simulink model "katayamacopter_r2021b"  (R2021b)
settings: Solver=VariableStepAuto  StartTime=0.0  StopTime=50  RelTol=1e-3
values from neighbouring files (symbols this model uses):
  A_pitch = [0  1; 0  0]    [param.mat]
  A_travel = [0  1; 0  -0.0247]    [param.mat]
  B_elev = [0  0; 0.655  0]    [param.mat]
  B_pitch = [0  0; 0  0.248]    [param.mat]
  B_travel = [0  0; 0.0086  0]    [param.mat]
  C_pitch = [1  0; 0  0]    [param.mat]
  C_travel = [1  0; 0  0]    [param.mat]
  D_elev = [0  0; 0  0]    [param.mat]
  D_pitch = [0  0; 0  0]    [param.mat]
  D_travel = [0  0; 0  0]    [param.mat]
libraries: robotlib x5, mpclib x3
settings Model: VariantFading=off  Creator=marik  LastModifiedBy=marik
settings DebuggingCC: UnconnectedInputMsg=none  UnconnectedOutputMsg=none  UnconnectedLineMsg=none  UnderSpecifiedDimensionMsg=warning
settings RTWCC: DLArmComputeVersion=20.02.1

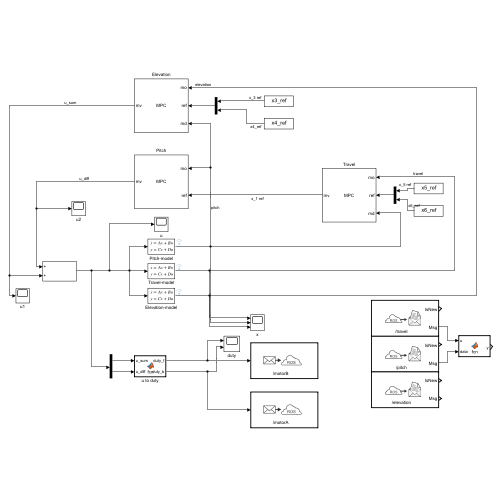
[thumbnail: Simulink's stored preview of the top-level diagram]
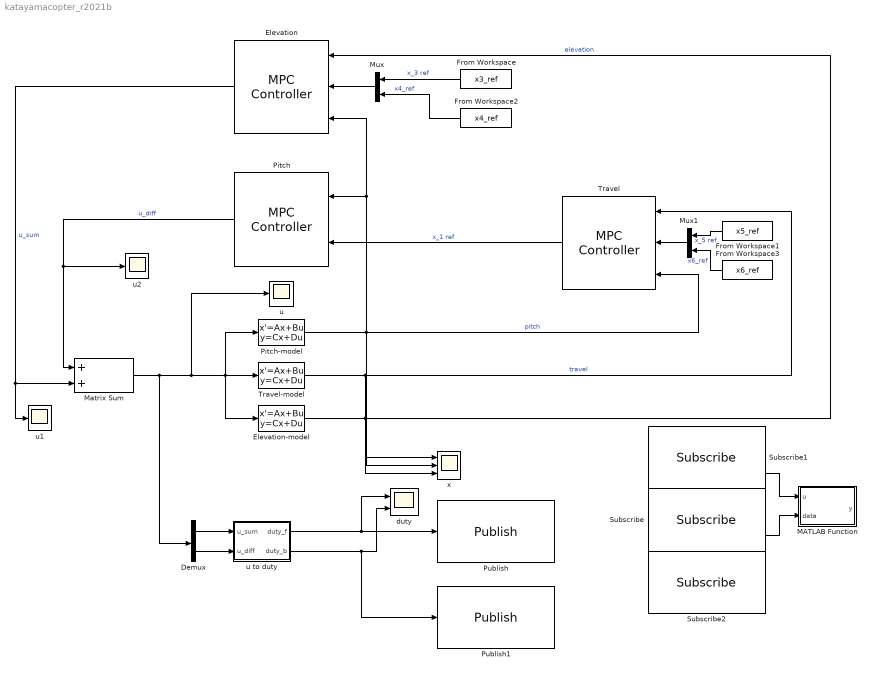
== system katayamacopter_r2021b ==
  Demux : Demux  Outputs=2
  Elevation : mpclib/MPC Controller  SCDEnableBlockLinearizationSpecification=on  mpcobj=mpcelev  is_multiple=0  enable_value=0  return_u0=off  updateMPCinCallerWorkspace=on  md_inport=on  mv_inport=off  uref_inport=off  return_cost=off  return_mvseq=off  return_qpstatus=off  return_xseq=off  return_state=off  return_ovseq=off  state_inport=off  umin_inport=off  umax_inport=off  ymin_inport=off  ymax_inport=off  cc_inport=off  ywt_inport=off  uwt_inport=off  duwt_inport=off  rhoeps_inport=off  pm_inport=off  MaximumP=10  HorizonChoice=FixedHorizon  n_ts=0.1  n_p=10  n_mv=2  n_md=1  n_ud=0  n_mo=2  n_uo=0  BlockDataType=double  SampleTimeInherited=off  switch_inport=off
  Elevation-model : StateSpace  A=[0 1;-1.283 -0.11]  B=B_elev  C=[1 0;0 1]  D=D_elev  InitialCondition=0
  From Workspace : FromWorkspace  VariableName=x3_ref  SampleTime=0.1  OutputAfterFinalValue=Holding final value
  From Workspace1 : FromWorkspace  VariableName=x5_ref  SampleTime=0.1  OutputAfterFinalValue=Holding final value
  From Workspace2 : FromWorkspace  VariableName=x4_ref
  From Workspace3 : FromWorkspace  VariableName=x6_ref
  MATLAB Function : MATLAB Function  TreatAsAtomicUnit=on
  Matrix Sum : Sum
  Mux : Mux  Inputs=2
  Mux1 : Mux  Inputs=2
  Pitch : mpclib/MPC Controller  SCDEnableBlockLinearizationSpecification=on  mpcobj=mpcpitch  is_multiple=0  enable_value=0  return_u0=off  updateMPCinCallerWorkspace=on  md_inport=off  mv_inport=off  uref_inport=off  return_cost=off  return_mvseq=off  return_qpstatus=off  return_xseq=off  return_state=off  return_ovseq=off  state_inport=off  umin_inport=off  umax_inport=off  ymin_inport=off  ymax_inport=off  cc_inport=off  ywt_inport=off  uwt_inport=off  duwt_inport=off  rhoeps_inport=off  pm_inport=off  MaximumP=10  HorizonChoice=FixedHorizon  n_ts=0.1  n_p=10  n_mv=2  n_md=0  n_ud=0  n_mo=2  n_uo=0  BlockDataType=double  SampleTimeInherited=off  switch_inport=off
  Pitch-model : StateSpace  A=A_pitch  B=B_pitch  C=C_pitch  D=D_pitch  InitialCondition=0
  Publish : robotlib/Publish  topicSource=Specify your own  topic=/motorB  messageType=std_msgs/Float32  legacyBusStruct=off  messageQueueLength=1
  Publish1 : robotlib/Publish  topicSource=Specify your own  topic=/motorA  messageType=std_msgs/Float32MultiArray  legacyBusStruct=off  messageQueueLength=1
  Subscribe : robotlib/Subscribe  topicSource=Specify your own  topic=/pitch  messageType=geometry_msgs/Point  SampleTime=-1  legacyBusStruct=off  messageQueueLength=1
  Subscribe1 : robotlib/Subscribe  topicSource=Specify your own  topic=/travel  messageType=std_msgs/Float32  SampleTime=-1  legacyBusStruct=off  messageQueueLength=1
  Subscribe2 : robotlib/Subscribe  topicSource=Specify your own  topic=/elevation  messageType=geometry_msgs/Point  SampleTime=-1  legacyBusStruct=off  messageQueueLength=1
  Travel : mpclib/MPC Controller  SCDEnableBlockLinearizationSpecification=on  mpcobj=mpctravel  is_multiple=0  enable_value=0  return_u0=off  updateMPCinCallerWorkspace=on  md_inport=on  mv_inport=off  uref_inport=off  return_cost=off  return_mvseq=off  return_qpstatus=off  return_xseq=off  return_state=off  return_ovseq=off  state_inport=off  umin_inport=off  umax_inport=off  ymin_inport=off  ymax_inport=off  cc_inport=off  ywt_inport=off  uwt_inport=off  duwt_inport=off  rhoeps_inport=off  pm_inport=off  MaximumP=10  HorizonChoice=FixedHorizon  n_ts=0.1  n_p=10  n_mv=2  n_md=1  n_ud=0  n_mo=2  n_uo=0  BlockDataType=double  SampleTimeInherited=off  switch_inport=off
  Travel-model : StateSpace  A=A_travel  B=B_travel  C=C_travel  D=D_travel  InitialCondition=0
  duty : Scope  NumInputPorts=2
  u : Scope
  u to duty : MATLAB Function  TreatAsAtomicUnit=on
  u1 : Scope
  u2 : Scope
  x : Scope  NumInputPorts=3
  wires:
  Travel/1 -> Pitch/2  "x_1 ref"
  From Workspace/1 -> Mux/1  "x_3 ref"
  Elevation-model/1 -> x/1, Elevation/1  "elevation"
  Pitch-model/1 -> x/2, Travel/3, Elevation/3, Pitch/1  "pitch"
  Travel-model/1 -> x/3, Travel/1  "travel"
  From Workspace1/1 -> Mux1/1  "x_5 ref"
  Elevation/1 -> u1/1, Matrix Sum/2  "u_sum"
  Pitch/1 -> u2/1, Matrix Sum/1  "u_diff"
  Matrix Sum/1 -> Demux/1, u/1, Pitch-model/1, Travel-model/1, Elevation-model/1
  From Workspace2/1 -> Mux/2  "x4_ref"
  Mux/1 -> Elevation/2
  Mux1/1 -> Travel/2
  From Workspace3/1 -> Mux1/2  "x6_ref"
  Demux/1 -> u to duty/1(u_sum)
  Demux/2 -> u to duty/2(u_diff)
  u to duty/1(duty_f) -> Publish/1, duty/1
  u to duty/2(duty_b) -> Publish1/1, duty/2
  Subscribe/2 -> MATLAB Function/2(data)
  Subscribe1/2 -> MATLAB Function/1(u)

== matlab function katayamacopter_r2021b/u to duty ==
  data: u_sum input; duty_f output; u_diff input; duty_b output
function [duty_f , duty_b] = fcn(u_sum,u_diff)
%sum/diff to forword/back
% u_sum = u_f + u_b
% u_diff = u_f - u_b
% ∴
% u_f = (u_sum + u_diff) / 2
% u_b = (u_sum - u_diff) / 2

u_f = (u_sum + u_diff) / 2;
u_b = (u_sum - u_diff) / 2;

%%
%u to duty
% 数値は片山の卒論fig4.3
duty_f = (u_f + 3.3235) / 0.6386;
duty_b = (u_b + 3.7394) / 0.7158;

== matlab function katayamacopter_r2021b/MATLAB Function ==
  data: u input; y output; data input
function y = fcn(u, data)

y = u;
